simulink model "p1"  (R2022b)
settings: Solver=VariableStepAuto  StartTime=0.0  StopTime=tsim  RelTol=1e-3
values from neighbouring files (symbols this model uses):
  rb = 1000    [p1_matlab.m]    (also in p2_matlab.m; p3_matlab.m; parte1.m; parte2.m)
  Spb = 10    [p1_matlab.m]    (also in p2_matlab.m = 100; p3_matlab.m = 100; parte1.m = 100; parte2.m = 100)
libraries: commchan3 x1, commrandsrc3 x1, dspsigops x1, commutil2 x1
settings Model: Creator=pedro  LastModifiedBy=joaogaspar
settings SolverCC: AlgebraicLoopSolver=TrustRegion
settings DebuggingCC: UnconnectedInputMsg=warning  UnconnectedOutputMsg=warning  UnconnectedLineMsg=warning  SFMachineParentedDataDiag=warning
settings ModelReferenceCC: EnableRefExpFcnMdlSchedulingChecks=on

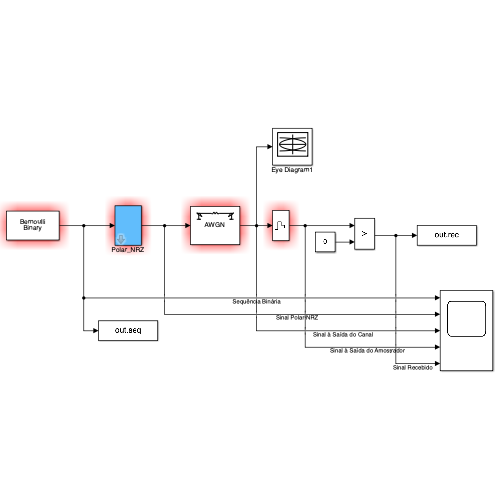
[thumbnail: Simulink's stored preview of the top-level diagram]
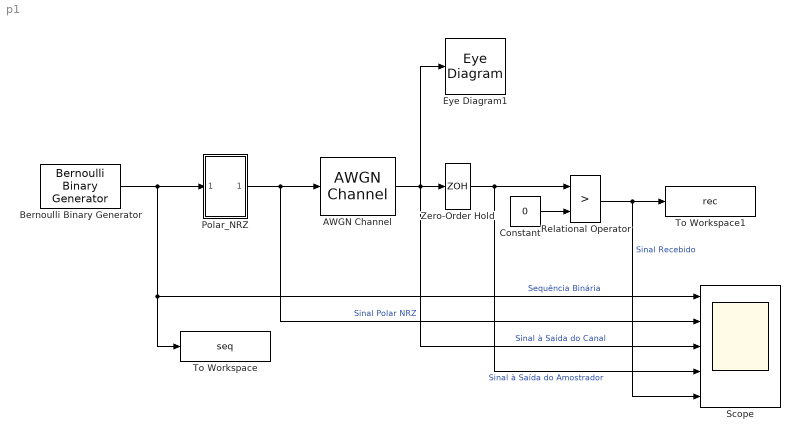
== system p1 ==
  AWGN Channel : commchan3/AWGN Channel  InputProcessing=Columns as channels (frame based)  seed=0  noiseMode=Variance from mask  EbNodB=10  EsNodB=10  SNRdB=10  bitsPerSym=1  Ps=1  Tsym=1  variance=sigmaquadrado
  Bernoulli Binary Generator : commrandsrc3/Bernoulli Binary Generator  ProbabilityOfZero=0.5  SeedSource=Parameter  Seed=0  SampleTime=1/rb  SamplesPerFrame=1  OutputDataType=double  SimulateUsing=Interpreted execution
  Constant : Constant  Value=0
  Eye Diagram1 : EyeDiagram
  Polar_NRZ : Subsystem  mask(Polar_nrz){Rb=rb, Spb=Spb}
      mask prompts: Rb "Binary Data Rate"; Spb "Samples per bit"
  Relational Operator : RelationalOperator  Operator=>  OutDataTypeStr=boolean  RndMeth=Simplest  InputSameDT=off
  Scope : Scope  NumInputPorts=5
  To Workspace : ToWorkspace  VariableName=seq  SaveFormat=Timeseries  SampleTime=-1
  To Workspace1 : ToWorkspace  VariableName=rec  SaveFormat=Timeseries  SampleTime=-1
  Zero-Order Hold : ZeroOrderHold  SampleTime=1/rb
  wires:
  Constant/1 -> Relational Operator/2
  AWGN Channel/1 -> Scope/3, Eye Diagram1/1, Zero-Order Hold/1  "Sinal à Saída do Canal"
  Polar_NRZ/1(Out1) -> Scope/2, AWGN Channel/1  "Sinal Polar NRZ"
  Bernoulli Binary Generator/1 -> To Workspace/1, Scope/1, Polar_NRZ/1(In1)  "Sequência Binária"
  Relational Operator/1 -> Scope/5, To Workspace1/1  "Sinal Recebido"
  Zero-Order Hold/1 -> Scope/4, Relational Operator/1  "Sinal à Saída do Amostrador"

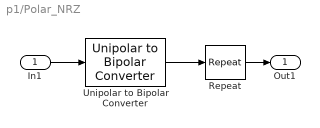
== system p1/Polar_NRZ ==
  In1 : Inport
  Repeat : dspsigops/Repeat  N=Spb  InputProcessing=Columns as channels (frame based)  RateOptions=Allow multirate processing  ic=0  mode=Unused parameter value
  Unipolar to Bipolar Converter : commutil2/Unipolar to Bipolar Converter  M=2  polarity=Positive  dataType=Same as input
  Out1 : Outport
  wires:
  Unipolar to Bipolar Converter/1 -> Repeat/1
  In1/1 -> Unipolar to Bipolar Converter/1
  Repeat/1 -> Out1/1
